simulink model "Laborator_1_simulink"  (R2022a)
settings: Solver=VariableStepAuto  StartTime=0.0  StopTime=300.0  RelTol=1e-3
libraries: simulink x1
settings Model: Creator=Petrisor  LastModifiedBy=Student
settings DebuggingCC: UnconnectedInputMsg=warning  UnconnectedOutputMsg=warning  UnconnectedLineMsg=warning
settings RTWCC: DLArmComputeVersion=19.05

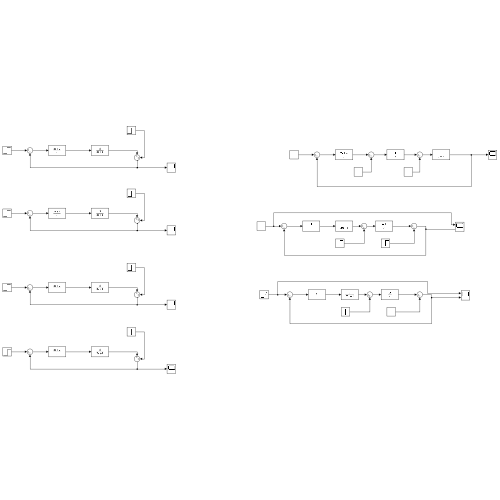
[thumbnail: Simulink's stored preview of the top-level diagram]
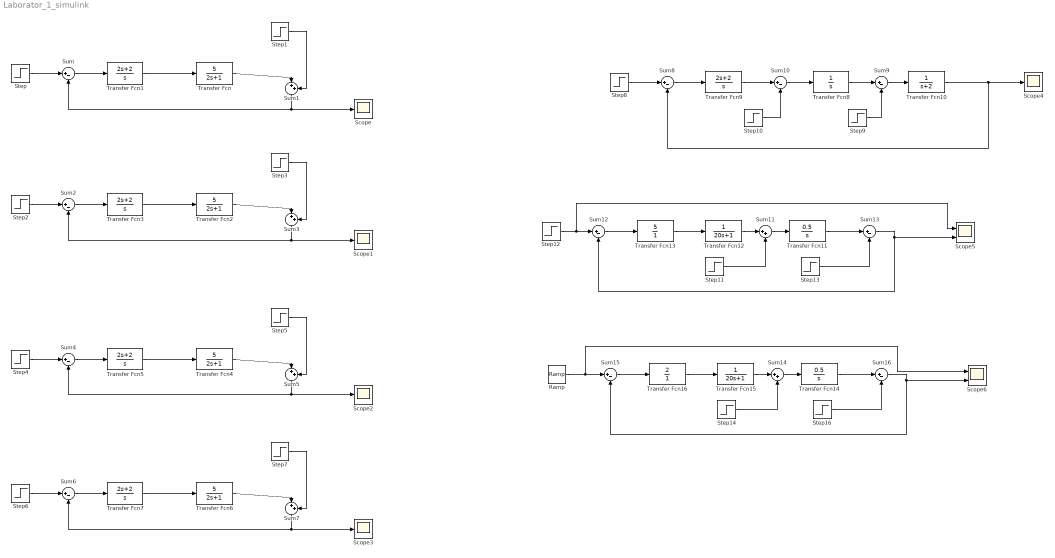
== system Laborator_1_simulink ==
  Ramp : simulink/Sources/Ramp  slope=1  start=0  InitialOutput=0
  Scope{,1..4} (5 alike) : Scope
  Scope5 : Scope  NumInputPorts=2
  Scope6 : Scope  NumInputPorts=2
  Step{,2,4,6,8,12} (6 alike) : Step  SampleTime=0
  Step1 : Step  After=0.5  SampleTime=0
  Step10 : Step  Time=0.1  After=0.7  SampleTime=0
  Step11 : Step  Time=0.2  After=0.2  SampleTime=0
  Step13 : Step  Time=0.2  After=0.1  SampleTime=0
  Step14 : Step  Time=0.1  After=0.1  SampleTime=0
  Step16 : Step  Time=0.2  After=0.1  SampleTime=0
  Step3 : Step  Time=0.2  SampleTime=0
  Step5 : Step  Time=0.3  SampleTime=0
  Step7 : Step  Time=0.4  SampleTime=0
  Step9 : Step  Time=0.6  After=0.5  SampleTime=0
  Sum{,2,4,6,8..10,12..13,15..16} (11 alike) : Sum  Inputs=|+-
  Sum{1,3,5,7,11,14} (6 alike) : Sum  Inputs=|++
  Transfer Fcn{,2,4,6} (4 alike) : TransferFcn  Numerator=[5]  Denominator=[2 1]
  Transfer Fcn{1,3,5,7,9} (5 alike) : TransferFcn  Numerator=[2 2]  Denominator=[1 0]
  Transfer Fcn10 : TransferFcn  Denominator=[1 2]
  Transfer Fcn11 : TransferFcn  Numerator=[0.5]  Denominator=[1 0]
  Transfer Fcn12 : TransferFcn  Denominator=[20 1]
  Transfer Fcn13 : TransferFcn  Numerator=[5]  Denominator=[1]
  Transfer Fcn14 : TransferFcn  Numerator=[0.5]  Denominator=[1 0]
  Transfer Fcn15 : TransferFcn  Denominator=[20 1]
  Transfer Fcn16 : TransferFcn  Numerator=[2]  Denominator=[1]
  Transfer Fcn8 : TransferFcn  Denominator=[1 0]
  wires:
  Transfer Fcn1/1 -> Transfer Fcn/1
  Step/1 -> Sum/1
  Sum/1 -> Transfer Fcn1/1
  Transfer Fcn/1 -> Sum1/1
  Sum1/1 -> Sum/2, Scope/1
  Step1/1 -> Sum1/2
  Transfer Fcn2/1 -> Sum3/1
  Sum3/1 -> Sum2/2, Scope1/1
  Transfer Fcn3/1 -> Transfer Fcn2/1
  Step2/1 -> Sum2/1
  Sum2/1 -> Transfer Fcn3/1
  Step3/1 -> Sum3/2
  Transfer Fcn4/1 -> Sum5/1
  Sum5/1 -> Sum4/2, Scope2/1
  Transfer Fcn5/1 -> Transfer Fcn4/1
  Step4/1 -> Sum4/1
  Sum4/1 -> Transfer Fcn5/1
  Step5/1 -> Sum5/2
  Transfer Fcn6/1 -> Sum7/1
  Sum7/1 -> Sum6/2, Scope3/1
  Transfer Fcn7/1 -> Transfer Fcn6/1
  Step6/1 -> Sum6/1
  Sum6/1 -> Transfer Fcn7/1
  Step7/1 -> Sum7/2
  Step8/1 -> Sum8/1
  Sum8/1 -> Transfer Fcn9/1
  Transfer Fcn9/1 -> Sum10/1
  Step10/1 -> Sum10/2
  Sum10/1 -> Transfer Fcn8/1
  Transfer Fcn8/1 -> Sum9/1
  Sum9/1 -> Transfer Fcn10/1
  Step9/1 -> Sum9/2
  Transfer Fcn10/1 -> Sum8/2, Scope4/1
  Step12/1 -> Scope5/1, Sum12/1
  Sum12/1 -> Transfer Fcn13/1
  Transfer Fcn13/1 -> Transfer Fcn12/1
  Transfer Fcn12/1 -> Sum11/1
  Step11/1 -> Sum11/2
  Sum11/1 -> Transfer Fcn11/1
  Transfer Fcn11/1 -> Sum13/1
  Step13/1 -> Sum13/2
  Sum13/1 -> Sum12/2, Scope5/2
  Transfer Fcn14/1 -> Sum16/1
  Sum14/1 -> Transfer Fcn14/1
  Step16/1 -> Sum16/2
  Sum15/1 -> Transfer Fcn16/1
  Sum16/1 -> Sum15/2, Scope6/2
  Transfer Fcn15/1 -> Sum14/1
  Step14/1 -> Sum14/2
  Transfer Fcn16/1 -> Transfer Fcn15/1
  Ramp/1 -> Scope6/1, Sum15/1
